simulink model "LAB2_2"  (R2020b)
settings: Solver=FixedStepDiscrete  StartTime=0.0  StopTime=30  FixedStep=0.0001  RelTol=1e-3
undefined symbols (not defined in the file): Ao, Bo, Co, DiscIntNeverNeededParam, Do, Fo, Go, Ho, K_e, K_I, National_Instruments, Nu, Nx, PCI, rpm2rads, sens, Ts
libraries: sldrtlib x3, simulink x1
settings Model: ExtModeTrigDuration=10001  Creator=umbe  LastModifiedBy=giorgiadisaro
settings HardwareCC: ProdBitPerLong=64  ProdHWDeviceType=Intel->x86-64 (Mac OS X)
settings RTWCC: Description=Simulink Desktop Real-Time  SystemTargetFile=sldrt.tlc  TemplateMakefile=sldrt.tmf  RTWCompilerOptimization=on
settings CodeAppCC: MaxIdLength=95
settings SimulinkDesktopRealTimeCC: TargetPreCompLibLocation=/Applications/MATLAB_R2020b.app/toolbox/sldrt/lib/maci64

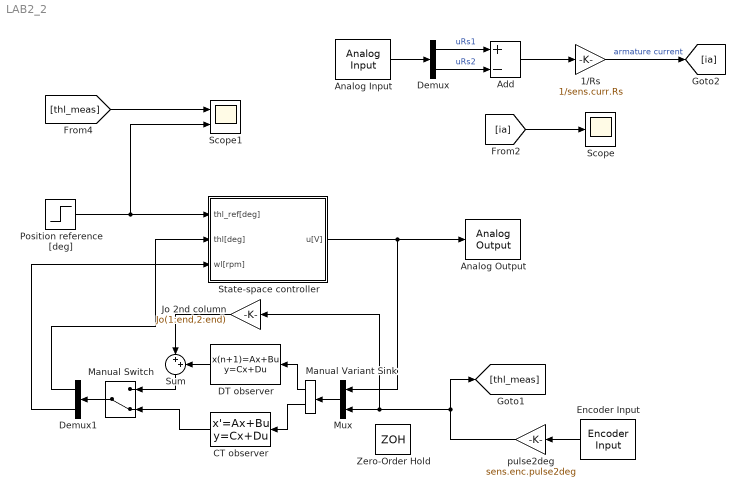
== system LAB2_2 ==
  1/Rs : Gain  Gain=1/sens.curr.Rs
  Add : Sum  Inputs=+-
  Analog Input : sldrtlib/Analog Input  SampleTime=-1  MaxMissedTicks=10  ShowMissedTicks=off  YieldWhenWaiting=off  DrvName=National_Instruments/PCI-6221  DrvAddress=4294967295  DrvOptions=[0 0 0 2 0]  Channels=[1 2]  RangeMode=1  VoltRange=1  DataType=1
      settings: AttributesFormatString=National Instruments\nPCI-6221 [auto]
  Analog Output : sldrtlib/Analog Output  SampleTime=-1  MaxMissedTicks=10  ShowMissedTicks=off  YieldWhenWaiting=off  DrvName=National_Instruments/PCI-6221  DrvAddress=4294967295  DrvOptions=[0 0 0 2 0]  Channels=1  RangeMode=1  VoltRange=1  InitialValue=0  FinalValue=0
      settings: AttributesFormatString=National Instruments\nPCI-6221 [auto]
  CT observer : StateSpace  A=Ao  B=Bo  C=Co  D=Do  InitialCondition=0
  DT observer : DiscreteStateSpace  A=Fo  B=Go  C=Ho  D=zeros(2,2)  SampleTime=Ts
  Demux : Demux  Outputs=2
  Demux1 : Demux  Outputs=2
  Encoder Input : sldrtlib/Encoder Input  SampleTime=-1  MaxMissedTicks=10  ShowMissedTicks=off  YieldWhenWaiting=off  DrvName=National_Instruments/PCI-6221  DrvAddress=4294967295  DrvOptions=[0 0 0 2 0]  Channels=1  QuadMode=3  IndexPulse=1  InputFilter=Inf  DataType=1
      settings: AttributesFormatString=National Instruments\nPCI-6221 [auto]
  Jo 2nd column : Gain  Gain=Jo(1:end,2:end)
  Manual Variant Sink : simulink/Signal Routing/Manual Variant Sink  NumChoices=2  LabelModeActiveChoice=V_2
  Manual Switch : ManualSwitch  CurrentSetting=0
  Mux : Mux  Inputs=2
  Position reference [deg] : Step  After=120  SampleTime=Ts
  Scope : Scope
  Scope1 : Scope  NumInputPorts=2
  State-space controller : Subsystem
  Sum : Sum  Inputs=|++
  Zero-Order Hold : ZeroOrderHold  SampleTime=Ts
  pulse2deg : Gain  Gain=sens.enc.pulse2deg
  wires:
  1/Rs/1 -> [ia]  "armature current"
  Add/1 -> 1/Rs/1
  Demux/1 -> Add/1  "uRs1"
  Demux/2 -> Add/2  "uRs2"
  [ia] -> Scope/1
  [thl_meas] -> Scope1/1
  Encoder Input/1 -> pulse2deg/1
  Analog Input/1 -> Demux/1
  pulse2deg/1 -> Jo 2nd column/1, Mux/2, [thl_meas]
  Demux1/1 -> State-space controller/2(thl[deg])
  Position reference [deg]/1 -> State-space controller/1(thl_ref[deg]), Scope1/2
  Demux1/2 -> State-space controller/3(wl[rpm])
  State-space controller/1(u[V]) -> Analog Output/1, Mux/1
  Manual Switch/1 -> Demux1/1
  CT observer/1 -> Manual Switch/2
  Mux/1 -> Manual Variant Sink/1
  Manual Variant Sink/1 -> DT observer/1
  Manual Variant Sink/2 -> CT observer/1
  Jo 2nd column/1 -> Sum/1
  DT observer/1 -> Sum/2
  Sum/1 -> Manual Switch/1

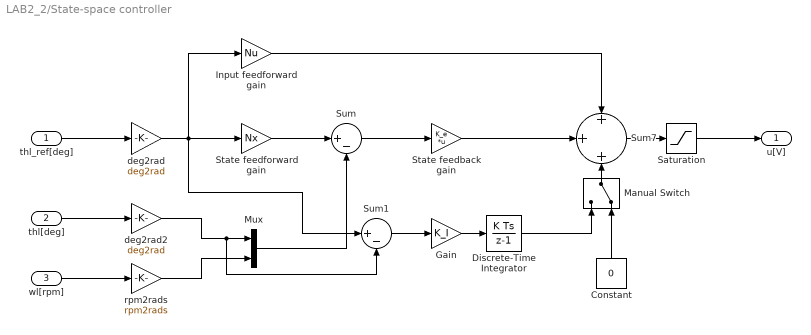
== system LAB2_2/State-space controller ==
  thl_ref[deg] : Inport
  thl[deg] : Inport  Port=2
  wl[rpm] : Inport  Port=3
  Constant : Constant  Value=0
  Discrete-Time Integrator : DiscreteIntegrator  SampleTime=Ts  ICPrevOutput=DiscIntNeverNeededParam  ICPrevScaledInput=DiscIntNeverNeededParam
  Gain : Gain  Gain=K_I
  Input feedforward gain : Gain  Gain=Nu
  Manual Switch : ManualSwitch  CurrentSetting=0
  Mux : Mux  Inputs=2
  Saturation : Saturate  UpperLimit=12  LowerLimit=-12
  "State feedback gain " : Gain  Gain=K_e  Multiplication=Matrix(K*u)
  State feedforward gain : Gain  Gain=Nx
  Sum : Sum  Inputs=|+-
  Sum1 : Sum  Inputs=|+-
  Sum7 : Sum  Inputs=+||+||+
  deg2rad : Gain  Gain=deg2rad
  deg2rad2 : Gain  Gain=deg2rad
  rpm2rads : Gain  Gain=rpm2rads
  u[V] : Outport
  wires:
  wl[rpm]/1 -> rpm2rads/1
  State feedforward gain/1 -> Sum/1
  deg2rad/1 -> Sum1/1, Input feedforward gain/1, State feedforward gain/1
  Sum/1 -> "State feedback gain "/1
  deg2rad2/1 -> Sum1/2, Mux/1
  Sum1/1 -> Gain/1
  thl[deg]/1 -> deg2rad2/1
  Gain/1 -> Discrete-Time Integrator/1
  Sum7/1 -> Saturation/1
  "State feedback gain "/1 -> Sum7/2
  Saturation/1 -> u[V]/1
  thl_ref[deg]/1 -> deg2rad/1
  Mux/1 -> Sum/2
  rpm2rads/1 -> Mux/2
  Input feedforward gain/1 -> Sum7/1
  Manual Switch/1 -> Sum7/3
  Discrete-Time Integrator/1 -> Manual Switch/1
  Constant/1 -> Manual Switch/2
